simulink model "MORUS_NELINEARNI_NELINEARNI_MPC"  (R2019a)
settings: Solver=FixedStepAuto  StartTime=0.0  StopTime=sim_time  RelTol=1e-3  EnableMultiTasking=on
values from neighbouring files (symbols this model uses):
  A_dis_calc = expm(kSamplingTime*A_continous_time)    [MPC_designer_X.m]    (also in NonTilting.m; RUN_simulation.m; Simulacija_MPC_YAW_NELINEARNI.m; Simulacija_MPC_Z.m)
  B_dis_calc = integral_exp_A * B_continous_time    [MPC_designer_X.m]    (also in NonTilting.m; RUN_simulation.m; Simulacija_MPC_YAW_NELINEARNI.m; Simulacija_MPC_Z.m)
  b_f = 4.56e-4    (= 0.000456)    [LinearizacijaMatrica.m]    (also in Linearizirane_matrice.mat; MPC_designer_X.m; NonTilting.m; RUN_simulation.m)
  b_m = 0.01    [LinearizacijaMatrica.m]    (also in Linearizirane_matrice.mat; MPC_designer_X.m; NonTilting.m; RUN_simulation.m)
  BETA = 0.0    (= 0)    [LinearizacijaMatrica.m]    (also in Linearizirane_matrice.mat; MPC_designer_X.m; NonTilting.m = 0.200712863979; RUN_simulation.m)
  g = 9.80665    [LinearizacijaMatrica.m]    (also in Linearizirane_matrice.mat; MPC_designer_X.m = 9.81; NonTilting.m = 9.81; RUN_simulation.m = 9.81)
  hover = 427.6233    [MPC_designer_X.m]    (also in NonTilting.m; RUN_simulation.m; Simulacija_MPC_YAW_NELINEARNI.m; Simulacija_MPC_Z.m)
  I_b_xx = 5.5268    [MPC_designer_X.m]    (also in NonTilting.m; RUN_simulation.m; Simulacija_MPC_YAW_NELINEARNI.m; Simulacija_MPC_Z.m)
  I_b_yy = 5.5268    [MPC_designer_X.m]    (also in NonTilting.m; RUN_simulation.m; Simulacija_MPC_YAW_NELINEARNI.m; Simulacija_MPC_Z.m)
  I_b_zz = 6.8854    [MPC_designer_X.m]    (also in NonTilting.m; RUN_simulation.m; Simulacija_MPC_YAW_NELINEARNI.m; Simulacija_MPC_Z.m)
  kSamplingTime = 0.810    (= 0.81)    [MPCDesigner_YAW.m]    (also in MPC_designer_X.m = 0.1; MPC_designer_Z.m; NonTilting.m = 0.015; RUN_simulation.m = 0.015)
  L = 0.84    [LinearizacijaMatrica.m]    (also in Linearizirane_matrice.mat; MPC_designer_X.m; NonTilting.m; RUN_simulation.m)
  m = 1.0    (= 1)    [LinearizacijaMatrica.m]    (also in Linearizirane_matrice.mat; MPC_designer_X.m; NonTilting.m; RUN_simulation.m)
  M = 34.8    [LinearizacijaMatrica.m]    (also in Linearizirane_matrice.mat; MPC_designer_X.m = 34; NonTilting.m = 34; RUN_simulation.m = 34)
  m_b = 30.8    [LinearizacijaMatrica.m]    (also in Linearizirane_matrice.mat; MPC_designer_X.m; NonTilting.m; RUN_simulation.m)
  odabir = 1    [MPC_designer_X.m]    (also in NonTilting.m; RUN_simulation.m; Simulacija_MPC_YAW_NELINEARNI.m; Simulacija_MPC_Z.m)
  polu = 1.0    (= 1)    [Simulacija_Roll.m]
  Q = inv(diag([0.5800 4*kSamplingTime 0.5800 4*kSamplingTime 300 300 0.2 (0.2/3) 100 4])) * diag([0, 0, 0, 0, 0, 0, 1e5,0, 1e7, 0]) *inv(diag([0.5800 4*kSamplingTime 0.5800 4*kSamplingTime 300 300 0.2 (0.2/3.0) 100 4]))    [NonTilting.m]    (also in RUN_simulation.m = diag([ 0.135340000000000,0.002706800000000,  0.1353400, 0.00; Simulacija_MPC_YAW_NELINEARNI.m = diag([pop(5),pop(6),pop(5),pop(6), pop(7),pop(7),pop(8),pop(; Simulacija_MPC_Z.m = diag([pop(5),pop(6),pop(5),pop(6), pop(7),pop(7),pop(8),pop(; Simulacija_Roll.m = diag([pop(5),pop(6),pop(5),pop(6), pop(7),pop(7),pop(8),pop()
  R = inv(diag([0.5800 0.5800 300 300]))*diag([0, 0, 0, 0])*inv(diag([0.5800 0.5800 300 300]))    [NonTilting.m]    (also in RUN_simulation.m = diag([0.67670, 0.67670, 0.13534000, 0.13534000]); Simulacija_MPC_YAW_NELINEARNI.m = diag([pop(1),pop(1),pop(2),pop(2)]); Simulacija_MPC_Z.m = diag([pop(1),pop(1),pop(2),pop(2)]); Simulacija_Roll.m = diag([pop(1),pop(1),pop(2),pop(2)]))
  R_delta = inv(diag([0.5800 0.5800 300 300]))* diag([0,0,0,0])*inv(diag([0.5800 0.5800 300 300]))    [NonTilting.m]    (also in RUN_simulation.m = diag([0.738879858135067, 0.738879858135067, 0.00738879858135; Simulacija_MPC_YAW_NELINEARNI.m = diag([pop(3),pop(3),pop(4),pop(4)]); Simulacija_MPC_Z.m = diag([pop(3),pop(3),pop(4),pop(4)]); Simulacija_Roll.m = diag([pop(3),pop(3),pop(4),pop(4)]))
  T_r = 0.2    [LinearizacijaMatrica.m]    (also in Linearizirane_matrice.mat; MPC_designer_X.m; NonTilting.m; RUN_simulation.m)
  w_mm = 19.7845    [LinearizacijaMatrica.m]    (also in Linearizirane_matrice.mat; MPC_designer_X.m = 17; NonTilting.m = 17; RUN_simulation.m = 17)
  z_m = 0.05    [LinearizacijaMatrica.m]    (also in Linearizirane_matrice.mat; MPC_designer_X.m; NonTilting.m; RUN_simulation.m)
  z_r = 0.2    [LinearizacijaMatrica.m]    (also in Linearizirane_matrice.mat; MPC_designer_X.m; NonTilting.m; RUN_simulation.m)
  zeta_mm = 0.6544    [LinearizacijaMatrica.m]    (also in Linearizirane_matrice.mat; MPC_designer_X.m = 0.85; NonTilting.m = 0.85; RUN_simulation.m = 0.85)
libraries: simulink x6
(part 5 of 5)

== matlab function MORUS_NELINEARNI_NELINEARNI_MPC/MPC PITCH/MATLAB Function3 ==
  settings: updateMethod=DISCRETE
  data: x0_ input; u output; x_ss_ input; u_ss_ input; kreni input; A input; B input; R input; R_delta input; Q input; samplingTime input
function u    = RMSProp(x0_, x_ss_, u_ss_, kreni, A, B, R, R_delta, Q, samplingTime)

persistent new_desire_state  pred_horizon control_horizon max_iter     ...
    scale_MV_inv   scale_OV_inv gradients gradient_past ...
    x_states deriv_wrt_u epsilon delta num_heuristic_vars ...
    u_past u_current lambdas_x lambdas_u lambdas_u_ref u_horizon ref_old t u_last_step ...
    du_max u_max  rho residuum_old 

residuum = 0;


if(isempty(new_desire_state) )
    residuum_old = 1e5;
    u_last_step = zeros(4, 1);
    du_max = zeros(4,2);
    u_max = zeros(4,2);
    
    du_max(1,1) = samplingTime * 2;
    du_max(1,2) = -samplingTime * 2;
    du_max(2,1) = samplingTime * 2;
    du_max(2,2) = -samplingTime * 2;
    du_max(3,1) = 1*(samplingTime/0.01);
    du_max(3,2) = -1*(samplingTime/0.01);
    du_max(4,1) = 1*(samplingTime/0.01);
    du_max(4,2) = -1*(samplingTime/0.01);
    rho = 0.999;
    u_max(1,1) = 0.6 / 2 - 0.01;
    u_max(1,2) = -u_max(1,1);
    u_max(2,1) = 0.6 / 2 - 0.01;
    u_max(2,2) = -u_max(1,1);
    u_max(3,1) = 50;
    u_max(3,2) = -50;
    u_max(4,1) = 50;
    u_max(4,2) = -50;
    
    ref_old  = x_ss_;
    t = 0.0;
    epsilon = 0.4;
    delta = 1e-7;
    max_iter = 15;
    control_horizon = 5;
    pred_horizon = 14;
    num_heuristic_vars = 2;
    gradients = zeros(num_heuristic_vars*control_horizon,1 );
    gradient_past = zeros(num_heuristic_vars*control_horizon,1 );
    new_desire_state = true;
    scale_OV_inv = inv(diag([0.58, 4.0, 0.58, 4.0, 800, 800, 0.5236, 0.5236]));
    
    scale_MV_inv = inv(diag([0.58, 0.58, 100, 100]));
%     
%     R =diag([0.67670, 0.67670, 0.13534000, 0.13534000]);
%     R_delta = diag([0.738879858135067, 0.738879858135067, 0.007388798581351,0.007388798581351]);
%     Q = diag([ 0.135340000000000,0.002706800000000,  0.1353400, 0.002706800, 0.002706800, 0.002706800,10.7068000, 9.676700]);
%     
%     A =[    0.4271,    0.0223,         0,         0,         0,         0,         0 ,        0;
%         -8.7243,   -0.1501,         0,         0,         0,         0,         0,         0;
%         0,         0,    0.4271,    0.0223,         0,         0,         0,         0;
%         0,         0,   -8.7243,   -0.1501,         0,         0,         0,         0;
%         0,         0,         0,         0,    0.7300,         0,         0,         0;
%         0,         0,         0,         0,         0,    0.7300,         0,         0;
%         0.0090,    0.0005,    0.0090,    0.0005,    0.0001,   -0.0001,    1.0000,    0.0787;
%         0.1699,    0.0113,    0.1699,    0.0113,    0.0028,   -0.0028,         0 ,   1.0000];
%     
%     B =[ 0.5729,         0 ,        0 ,        0;
%         8.7243,         0   ,      0 ,        0;
%         0,    0.5729  ,       0 ,        0;
%         0,    8.7243 ,        0 ,        0;
%         0,         0 ,   0.2700 ,        0;
%         0,         0 ,        0 ,   0.2700;
%         -0.0037,   -0.0037,    0.0000 ,  -0.0000;
%         -0.0347,   -0.0347,    0.0005 ,  -0.0005];
    
    
    
    x_states = zeros(size(A, 1), pred_horizon+1);
    deriv_wrt_u =  zeros(size(B,2), control_horizon);
    u_past = zeros(size(B,2), 1);
    u_current = zeros(size(B,2), 1);
    u_ss_ = zeros(size(B,2), 1);
    lambdas_x = zeros(size(A, 1), pred_horizon);
    lambdas_u = zeros(size(B,2), pred_horizon);
    u_horizon = zeros(size(B,2), pred_horizon);
    lambdas_u_ref = zeros(size(B,2), pred_horizon);
    
end

residuum_signal =0.0;
residuum_state =0.0;

u = zeros(size(B,2), 1);
if(kreni ~= 3)
    return
end
x = zeros(control_horizon *num_heuristic_vars,1);
change_x = zeros(control_horizon *num_heuristic_vars,1);

if(sum(sum(abs(x_ss_ - ref_old), 'double')) < 1e-6)
    new_desire_state = false;
    
else
    new_desire_state = true;
    ref_old = x_ss_;
end
if (new_desire_state)
        new_desire_state = false;
        gradient_past = 0*gradient_past;
        residuum_old = 1e5;
end

if(residuum_old < 1e-4)
    return;
end

for iter = 1:max_iter
    x_states(:,1) = x0_ ;
    deriv_wrt_u = 0*deriv_wrt_u;
    u_past = zeros(size(B,2), 1);% u_current*1;
    
    
    
    for i = 1:pred_horizon
        if(i <= control_horizon)
            u(1,1) = x(0*control_horizon  + i);
            u(2,1) = x(0*control_horizon  + i);
            u(3,1) = x(1*control_horizon  + i);
            u(4,1) = -x(1*control_horizon  + i);
        end
        x_states(:,i+1) = A * x_states(:,i) + B * u;
        lambdas_x(:,i) = -1*x_ss_ + x_states(:,i+1);
        lambdas_u(:,i) = u - u_past;
        lambdas_u_ref(:, i) = u - u_ss_;
        
        %derivation of u
        if(i <= control_horizon)
            deriv_wrt_u(:, i) = (2*R*u) -2*R*u_ss_  + (4*R_delta*u) -2*R_delta*u_past + deriv_wrt_u(:, i) ;
            
            if(i > 1)
                deriv_wrt_u(:, i-1) = deriv_wrt_u(:, i-1) -2*R_delta*u ;
            end
        else
            deriv_wrt_u(:, control_horizon) = deriv_wrt_u(:, control_horizon) + (2*R*u) -2*R*u_ss_  + (4*R_delta*u)+ (-2*R_delta*u_past) ;
            deriv_wrt_u(:, control_horizon) = deriv_wrt_u(:, control_horizon) -2*R_delta*u ;
        end
        
        %derivation of x
        for j = 1:i
            if(j <= control_horizon && i <= control_horizon)
                
                deriv_wrt_u(:,j) = deriv_wrt_u(:,j) + transpose(transpose( 2*Q*x_states(:,i+1) - 2*Q*x_ss_ )*(A^(i-j))*B);
            else
                if(j > control_horizon)
                    deriv_wrt_u(:,control_horizon) =deriv_wrt_u(:,control_horizon) +  transpose(transpose((2*Q*x_states(:,i+1) - 2*Q*x_ss_))*(A^(i-j))*B);
                else
                    deriv_wrt_u(:,j) =deriv_wrt_u(:,j) + transpose(transpose( 2*Q*x_states(:,i+1) - 2*Q*x_ss_ )*(A^(i-j))*B);
                end
            end
        end
        u_past = u;
    end
    
    
    lambdas_u_ref =scale_MV_inv * lambdas_u_ref;
    lambdas_u = scale_MV_inv * lambdas_u;
    lambdas_x = scale_OV_inv * lambdas_x;
    residuum_signal=sum(sum((lambdas_u_ref.*(R*lambdas_u_ref)),'double'))  + sum(sum((lambdas_u.*(R_delta*lambdas_u)),'double'));
    residuum_state=sum(sum((lambdas_x.*(Q*lambdas_x)),'double')) ;
    
    residuum =  residuum_signal +  residuum_state;
    
    
    
    for iter_der = 1:control_horizon
        gradients(iter_der, 1) = 2 * deriv_wrt_u(1, iter_der);
        gradients(iter_der + control_horizon, 1) = 2 * deriv_wrt_u(3, iter_der);
    end
    
    
    gradient_past = (rho*gradient_past + (1-rho)*gradients.*gradients);
    
    
    
    for adam_iter = 1:control_horizon *num_heuristic_vars
        change_x(adam_iter, 1) = -1 * (epsilon * gradients(adam_iter, 1)) / (sqrt(gradient_past(adam_iter, 1)) + delta);
        
    end
    
    x = (x + change_x);
end

u(1,1) = x(0*control_horizon  + 1);
u(2,1) = x(0*control_horizon  + 1);
u(3,1) = x(1*control_horizon  + 1);
u(4,1) = -x(1*control_horizon  + 1);

for iter_m = 1:4
    if(u(iter_m,1) > ( u_last_step(iter_m,1)+du_max(iter_m,1) ))
        u(iter_m,1) =  u_last_step(iter_m,1)+du_max(iter_m,1);
        
    elseif (u(iter_m,1) < ( u_last_step(iter_m,1)+du_max(iter_m,2) ))
        u(iter_m,1) =  u_last_step(iter_m,1)+du_max(iter_m,2);
    end
    
    if(u(iter_m,1) > u_max(iter_m,1) )
        u(iter_m,1) =  u_max(iter_m,1);
    elseif (u(iter_m,1) < u_max(iter_m,2))
        u(iter_m,1) =  u_max(iter_m,2);
    end
    
    
end
if(residuum_old < residuum)
    u = 0*u;
    return;
end
u_last_step = u;
residuum_old = residuum;
end

== matlab function MORUS_NELINEARNI_NELINEARNI_MPC/MPC PITCH/MATLAB Function4 ==
  settings: updateMethod=DISCRETE
  data: x0_ input; u output; x_ss_ input; u_ss_ input; kreni input; A input; B input; R input; R_delta input; Q input; samplingTime input
function u   = RMSPropNester(x0_, x_ss_, u_ss_, kreni, A, B, R, R_delta, Q, samplingTime)

persistent new_desire_state  pred_horizon control_horizon max_iter    ...
    scale_MV_inv   scale_OV_inv gradients gradient_past ...
    x_states deriv_wrt_u epsilon delta num_heuristic_vars ...
    u_past u_current lambdas_x lambdas_u lambdas_u_ref u_horizon ref_old t u_last_step ...
    du_max u_max  rho residuum_old alpha change_x x

residuum = 0;


if(isempty(new_desire_state) )
    residuum_old = 1e25;
    u_last_step = zeros(4, 1);
    du_max = zeros(4,2);
    u_max = zeros(4,2);
    alpha = 200;
    du_max(1,1) = samplingTime * 2;
    du_max(1,2) = -samplingTime * 2;
    du_max(2,1) = samplingTime * 2;
    du_max(2,2) = -samplingTime * 2;
    du_max(3,1) = 1*(samplingTime/0.01);
    du_max(3,2) = -1*(samplingTime/0.01);
    du_max(4,1) = 1*(samplingTime/0.01);
    du_max(4,2) = -1*(samplingTime/0.01);
    rho = 0.999;
    u_max(1,1) = 0.6 / 2 - 0.01;
    u_max(1,2) = -u_max(1,1);
    u_max(2,1) = 0.6 / 2 - 0.01;
    u_max(2,2) = -u_max(1,1);
    u_max(3,1) = 50;
    u_max(3,2) = -50;
    u_max(4,1) = 50;
    u_max(4,2) = -50;
    
    ref_old  = x_ss_;
    t = 0.0;
    epsilon = 0.4;
    delta = 1e-7;
    max_iter = 15;
    control_horizon = 5;
    pred_horizon = 14;
    num_heuristic_vars = 2;
    gradients = zeros(num_heuristic_vars*control_horizon,1 );
    gradient_past = zeros(num_heuristic_vars*control_horizon,1 );
    new_desire_state = true;
    scale_OV_inv = inv(diag([0.58, 4.0, 0.58, 4.0, 800, 800, 0.5236, 0.5236]));
    
    scale_MV_inv = inv(diag([0.58, 0.58, 100, 100]));
    
%     R =diag([0.67670, 0.67670, 0.13534000, 0.13534000]);
%     R_delta = diag([0.738879858135067, 0.738879858135067, 0.007388798581351,0.007388798581351]);
%     Q = diag([ 0.135340000000000,0.002706800000000,  0.1353400, 0.002706800, 0.002706800, 0.002706800,10.7068000, 9.676700]);
%     
%     A =[    0.4271,    0.0223,         0,         0,         0,         0,         0 ,        0;
%         -8.7243,   -0.1501,         0,         0,         0,         0,         0,         0;
%         0,         0,    0.4271,    0.0223,         0,         0,         0,         0;
%         0,         0,   -8.7243,   -0.1501,         0,         0,         0,         0;
%         0,         0,         0,         0,    0.7300,         0,         0,         0;
%         0,         0,         0,         0,         0,    0.7300,         0,         0;
%         0.0090,    0.0005,    0.0090,    0.0005,    0.0001,   -0.0001,    1.0000,    0.0787;
%         0.1699,    0.0113,    0.1699,    0.0113,    0.0028,   -0.0028,         0 ,   1.0000];
%     
%     B =[ 0.5729,         0 ,        0 ,        0;
%         8.7243,         0   ,      0 ,        0;
%         0,    0.5729  ,       0 ,        0;
%         0,    8.7243 ,        0 ,        0;
%         0,         0 ,   0.2700 ,        0;
%         0,         0 ,        0 ,   0.2700;
%         -0.0037,   -0.0037,    0.0000 ,  -0.0000;
%         -0.0347,   -0.0347,    0.0005 ,  -0.0005];
    
    
    
    x_states = zeros(size(A, 1), pred_horizon+1);
    deriv_wrt_u =  zeros(size(B,2), control_horizon);
    u_past = zeros(size(B,2), 1);
    u_current = zeros(size(B,2), 1);
    u_ss_ = zeros(size(B,2), 1);
    lambdas_x = zeros(size(A, 1), pred_horizon);
    lambdas_u = zeros(size(B,2), pred_horizon);
    u_horizon = zeros(size(B,2), pred_horizon);
    lambdas_u_ref = zeros(size(B,2), pred_horizon);
    change_x = zeros(control_horizon *num_heuristic_vars,1);
    x = zeros(control_horizon *num_heuristic_vars,1);

    
end

residuum_signal =0.0;
residuum_state =0.0;

u = zeros(size(B,2), 1);
if(kreni ~= 4)
    return
end
change_x = zeros(control_horizon *num_heuristic_vars,1);

if(sum(sum(abs(x_ss_ - ref_old), 'double')) < 1e-6)
    new_desire_state = false;
    
else
    new_desire_state = true;
    ref_old = x_ss_;
end
if (new_desire_state)
        new_desire_state = false;
        gradient_past = 0*gradient_past;
        residuum_old = 1e25;
        alpha = 200;
        x = zeros(control_horizon *num_heuristic_vars,1);

end

if(residuum_old < 1e-4)
    return;
end

for iter = 1:max_iter
    x_states(:,1) = x0_ ;
    deriv_wrt_u = 0*deriv_wrt_u;
    u_past = zeros(size(B,2), 1);% u_current*1;
    
    
    x_tilda = x + alpha * change_x;
    for i = 1:pred_horizon
        if(i <= control_horizon)
            u(1,1) = x_tilda(0*control_horizon  + i);
            u(2,1) = x_tilda(0*control_horizon  + i);
            u(3,1) = x_tilda(1*control_horizon  + i);
            u(4,1) = -x_tilda(1*control_horizon  + i);
        end
        x_states(:,i+1) = A * x_states(:,i) + B * u;
        lambdas_x(:,i) = -1*x_ss_ + x_states(:,i+1);
        lambdas_u(:,i) = u - u_past;
        lambdas_u_ref(:, i) = u - u_ss_;
        
        %derivation of u
        if(i <= control_horizon)
            deriv_wrt_u(:, i) = (2*R*u) -2*R*u_ss_  + (4*R_delta*u) -2*R_delta*u_past + deriv_wrt_u(:, i) ;
            
            if(i > 1)
                deriv_wrt_u(:, i-1) = deriv_wrt_u(:, i-1) -2*R_delta*u ;
            end
        else
            deriv_wrt_u(:, control_horizon) = deriv_wrt_u(:, control_horizon) + (2*R*u) -2*R*u_ss_  + (4*R_delta*u)+ (-2*R_delta*u_past) ;
            deriv_wrt_u(:, control_horizon) = deriv_wrt_u(:, control_horizon) -2*R_delta*u ;
        end
        
        %derivation of x
        for j = 1:i
            if(j <= control_horizon && i <= control_horizon)
                
                deriv_wrt_u(:,j) = deriv_wrt_u(:,j) + transpose(transpose( 2*Q*x_states(:,i+1) - 2*Q*x_ss_ )*(A^(i-j))*B);
            else
                if(j > control_horizon)
                    deriv_wrt_u(:,control_horizon) =deriv_wrt_u(:,control_horizon) +  transpose(transpose((2*Q*x_states(:,i+1) - 2*Q*x_ss_))*(A^(i-j))*B);
                else
                    deriv_wrt_u(:,j) =deriv_wrt_u(:,j) + transpose(transpose( 2*Q*x_states(:,i+1) - 2*Q*x_ss_ )*(A^(i-j))*B);
                end
            end
        end
        u_past = u;
    end
    
    
    lambdas_u_ref =scale_MV_inv * lambdas_u_ref;
    lambdas_u = scale_MV_inv * lambdas_u;
    lambdas_x = scale_OV_inv * lambdas_x;
    residuum_signal=sum(sum((lambdas_u_ref.*(R*lambdas_u_ref)),'double'))  + sum(sum((lambdas_u.*(R_delta*lambdas_u)),'double'));
    residuum_state=sum(sum((lambdas_x.*(Q*lambdas_x)),'double')) ;
    
    residuum =  residuum_signal +  residuum_state;
    if(residuum < 0.1)
        alpha = 1e-5;
    end
    
    
    for iter_der = 1:control_horizon
        gradients(iter_der, 1) = 2 * deriv_wrt_u(1, iter_der);
        gradients(iter_der + control_horizon, 1) = 2 * deriv_wrt_u(3, iter_der);
    end
    
    
    gradient_past = (rho*gradient_past + (1-rho)*gradients.*gradients);
    
    
    
    for adam_iter = 1:control_horizon *num_heuristic_vars
        change_x(adam_iter, 1) =alpha * change_x(adam_iter, 1)  -1 * (epsilon * gradients(adam_iter, 1)) / (sqrt(gradient_past(adam_iter, 1)) + delta);
        
    end
    
    x = (x + change_x);
end

u(1,1) = x(0*control_horizon  + 1);
u(2,1) = x(0*control_horizon  + 1);
u(3,1) = x(1*control_horizon  + 1);
u(4,1) = -x(1*control_horizon  + 1);

for iter_m = 1:4
    if(u(iter_m,1) > ( u_last_step(iter_m,1)+du_max(iter_m,1) ))
        u(iter_m,1) =  u_last_step(iter_m,1)+du_max(iter_m,1);
        
    elseif (u(iter_m,1) < ( u_last_step(iter_m,1)+du_max(iter_m,2) ))
        u(iter_m,1) =  u_last_step(iter_m,1)+du_max(iter_m,2);
    end
    
    if(u(iter_m,1) > u_max(iter_m,1) )
        u(iter_m,1) =  u_max(iter_m,1);
    elseif (u(iter_m,1) < u_max(iter_m,2))
        u(iter_m,1) =  u_max(iter_m,2);
    end
    
    
end
if(residuum_old < residuum)
    u = 0*u;
    return;
end
u_last_step = u;
residuum_old = residuum;
end

== matlab function MORUS_NELINEARNI_NELINEARNI_MPC/MATLAB Function ==
  data: OMEGA_1 input size=1; A_dis_calc output size=8,8; OMEGA_2 input size=1; OMEGA_3 input size=1; OMEGA_4 input size=1; DOT_YAW input size=1; ROLL input size=1; PITCH input size=1; DOT_PITCH input size=1; DOT_ROLL input size=1; x_1 input size=1; x_3 input size=1; y_2 input size=1; y_4 input size=1; DOT_x_1 input size=1; DOT_x_3 input size=1; DOT_y_2 input size=1; DOT_y_4 input size=1; x_1_ref input size=1; x_3_ref input size=1; y_2_ref input size=1; y_4_ref input size=1; kSamplingTime input size=1; B_dis_calc output size=8,4
function [A_dis_calc ,B_dis_calc] = getROLLMAT(OMEGA_1, OMEGA_2, OMEGA_3, OMEGA_4, DOT_YAW , ROLL, PITCH, DOT_PITCH, DOT_ROLL,  x_1, x_3, y_2, y_4, DOT_x_1 ,DOT_x_3 ,DOT_y_2, DOT_y_4, x_1_ref, x_3_ref, y_2_ref, y_4_ref, kSamplingTime)

kGravity = 9.80665;
mass_ = 1.0;
mass_quad_ = 30.8;
M_ = mass_quad_ + 4 * mass_;
mi_ = mass_ / M_;

zm_ = 0.05;

lm_ = 0.6;
 Iq_xx = 5.5268 + 0.2;
 Iq_yy = 5.5268 + 0.2;
 Iq_zz = 6.8854 + 0.4;
Iq_ = zeros(3, 3);
Iq_(1, 1) = Iq_xx;
Iq_(2, 2) = Iq_yy;
Iq_(3, 3) = Iq_zz;
Iyy_b_ = 5.5268;
Iyy_ = Iyy_b_ + 2 * mass_ * (lm_ / 2)^ 2;

Tgm_ = 0.25;
w_gm_n_ = 7000 / 60 * 2 * pi;
F_n_ = 25 * kGravity;
b_gm_f_ = F_n_ / (w_gm_n_^ 2);

w_gm_0_ = sqrt(M_ * kGravity / 4.0 / b_gm_f_);





zeta_mm_ = 0.6544;
w_mm_ = 19.7845;
A_continous_time = zeros(8,8);
A_continous_time(1+0, 1+ 1) = 1.0;
A_continous_time(1+1, 1+ 0) = -(w_mm_^ 2);
A_continous_time(1+1, 1+ 1) = -2.0 * zeta_mm_ * w_mm_;
A_continous_time(1+2, 1+ 3) = 1.0;
A_continous_time(1+3, 1+ 2) = -(w_mm_^  2);
A_continous_time(1+3, 1+ 3) = -2.0 * zeta_mm_ * w_mm_;
A_continous_time(1+4, 1+ 4) = -1.0 / Tgm_;
A_continous_time(1+5, 1+ 5) = -1.0 / Tgm_;
A_continous_time(1+6, 1+ 7) = 1.0;
A_continous_time(1+7, 1+ 0) = 1.0 * mass_ / Iyy_ * (kGravity + ((1.0 - 4.0 * mi_) * zm_ * (w_mm_^ 2)));
A_continous_time(1+7, 1+ 1) = 2.0 * mass_ * (1.0 - 4.0 * mi_) * zm_ * zeta_mm_ * w_mm_ / Iyy_;
A_continous_time(1+7, 1+ 2) = mass_ / Iyy_ * (kGravity + ((1.0 - 4.0 * mi_) * zm_ * (w_mm_^ 2)));
A_continous_time(1+7, 1+ 3) = 2.0 * mass_ * (1.0 - 4.0 * mi_) * zm_ * zeta_mm_ * w_mm_ / Iyy_;
A_continous_time(1+7, 1+ 4) = 2 * b_gm_f_ * w_gm_0_ * lm_ / Iyy_;
A_continous_time(1+7, 1+ 5) = -2 * b_gm_f_ * w_gm_0_ * lm_ / Iyy_;

B_continous_time = zeros(8,4);
B_continous_time(1+1, 1+ 0) = (w_mm_^ 2);
B_continous_time(1+3, 1+ 1) = (w_mm_^ 2);
B_continous_time(1+4, 1+ 2) = 1.0 / Tgm_;
B_continous_time(1+5, 1+ 3) = 1.0 / Tgm_;
B_continous_time(1+7, 1+ 0) =-(16569550015242945875*cos(ROLL))/(8796093022208*(105625*x_1^2 - 6250*x_1*x_3 + 91350*x_1 + 105625*x_3^2 - 91350*x_3 + 640369));
B_continous_time(1+7, 1+ 1) =-(16569550015242945875*cos(ROLL))/(8796093022208*(105625*x_1^2 - 6250*x_1*x_3 + 91350*x_1 + 105625*x_3^2 - 91350*x_3 + 640369));


A_continous_time(8,:) = [(108750*cos(ROLL)*((3504881374004815*OMEGA_1^2)/267477789068788498432 + (3504881374004815*OMEGA_2^2)/267477789068788498432 + (3504881374004815*OMEGA_3^2)/267477789068788498432 + (3504881374004815*OMEGA_4^2)/267477789068788498432 - (14318*DOT_x_1*(DOT_PITCH*cos(ROLL) + DOT_YAW*cos(PITCH)*sin(ROLL)))/7569 + (820*DOT_x_3*(DOT_PITCH*cos(ROLL) + DOT_YAW*cos(PITCH)*sin(ROLL)))/7569 - ((5*DOT_ROLL)/174 - (5*DOT_YAW*sin(PITCH))/174)*(DOT_y_2 + DOT_y_4) - ((385*DOT_x_1)/7569 + (385*DOT_x_3)/7569)*(DOT_PITCH*cos(ROLL) + DOT_YAW*cos(PITCH)*sin(ROLL)) - (DOT_ROLL - DOT_YAW*sin(PITCH))*(DOT_PITCH*sin(ROLL) - DOT_YAW*cos(PITCH)*cos(ROLL))*((169*x_1)/87 - (5*x_3)/87 + 21/25) + 132556400121943567/7652600929320960))/(105625*x_1^2 - 6250*x_1*x_3 + 91350*x_1 + 105625*x_3^2 - 91350*x_3 + 640369) - (87000*sin(ROLL)*((5*DOT_y_2)/174 + (5*DOT_y_4)/174 + (14318*DOT_x_1*(DOT_PITCH*sin(ROLL) - DOT_YAW*cos(PITCH)*cos(ROLL)))/7569 - (820*DOT_x_3*(DOT_PITCH*sin(ROLL) - DOT_YAW*cos(PITCH)*cos(ROLL)))/7569 + ((385*DOT_x_1)/7569 + (385*DOT_x_3)/7569)*(DOT_PITCH*sin(ROLL) - DOT_YAW*cos(PITCH)*cos(ROLL)) - (DOT_ROLL - DOT_YAW*sin(PITCH))*(DOT_PITCH*cos(ROLL) + DOT_YAW*cos(PITCH)*sin(ROLL))*((169*x_1)/87 - (5*x_3)/87 + 21/25)))/(84500*x_1^2 - 5000*x_1*x_3 + 73080*x_1 + 84500*x_3^2 - 73080*x_3 + 84500*y_2^2 - 5000*y_2*y_4 + 73080*y_2 + 84500*y_4^2 - 73080*y_4 + 660417) - (7569000000*sin(ROLL)*((169*x_1)/87 - (5*x_3)/87 + 21/25)*((1345874447617849*OMEGA_2^2)/295147905179352825856 + (1345874447617849*OMEGA_4^2)/295147905179352825856 + (DOT_PITCH*sin(ROLL) - DOT_YAW*cos(PITCH)*cos(ROLL))*((820*DOT_x_1*x_3)/7569 + (820*DOT_x_3*x_1)/7569 + (820*DOT_y_2*y_4)/7569 + (820*DOT_y_4*y_2)/7569) - (DOT_PITCH*sin(ROLL) - DOT_YAW*cos(PITCH)*cos(ROLL))*((14318*DOT_x_1*x_1)/7569 + (14318*DOT_x_3*x_3)/7569 + (14318*DOT_y_2*y_2)/7569 + (14318*DOT_y_4*y_4)/7569) + (DOT_ROLL - DOT_YAW*sin(PITCH))*((77*DOT_x_1)/1740 + (77*DOT_x_3)/1740) - (DOT_PITCH*sin(ROLL) - DOT_YAW*cos(PITCH)*cos(ROLL))*((21*DOT_x_1)/25 - (21*DOT_x_3)/25 + (21*DOT_y_2)/25 - (21*DOT_y_4)/25) - (5*(x_1 + x_3)*(DOT_y_2 + DOT_y_4))/174 + (5*(y_2 + y_4)*(DOT_x_1 + DOT_x_3))/174 - (1345874447617849*OMEGA_1^2)/295147905179352825856 - (1345874447617849*OMEGA_3^2)/295147905179352825856 - ((385*(x_1 + x_3)*(DOT_x_1 + DOT_x_3))/7569 + (385*(y_2 + y_4)*(DOT_y_2 + DOT_y_4))/7569)*(DOT_PITCH*sin(ROLL) - DOT_YAW*cos(PITCH)*cos(ROLL)) + ((77*DOT_y_2)/1740 + (77*DOT_y_4)/1740)*(DOT_PITCH*cos(ROLL) + DOT_YAW*cos(PITCH)*sin(ROLL)) + (DOT_ROLL - DOT_YAW*sin(PITCH))*(DOT_PITCH*cos(ROLL) + DOT_YAW*cos(PITCH)*sin(ROLL))*((169*x_1^2)/174 - (5*x_1*x_3)/87 + (21*x_1)/25 + (169*x_3^2)/174 - (21*x_3)/25 - (169*y_2^2)/174 + (5*y_2*y_4)/87 - (21*y_2)/25 - (169*y_4^2)/174 + (21*y_4)/25)))/(84500*x_1^2 - 5000*x_1*x_3 + 73080*x_1 + 84500*x_3^2 - 73080*x_3 + 84500*y_2^2 - 5000*y_2*y_4 + 73080*y_2 + 84500*y_4^2 - 73080*y_4 + 660417)^2 - (11826562500*cos(ROLL)*((169*x_1)/87 - (5*x_3)/87 + 21/25)*((187071499653674713*DOT_x_1)/163255486492180480 + (187071499653674713*DOT_x_3)/163255486492180480 + (132556400121943567*x_1)/7652600929320960 + (132556400121943567*x_3)/7652600929320960 - (132556400121943567*x_1_ref)/7652600929320960 - (132556400121943567*x_3_ref)/7652600929320960 + (2102928824402889*OMEGA_1^2*((5*x_1)/174 + (5*x_3)/174 - 21/25))/4611686018427387904 + (2102928824402889*OMEGA_3^2*((5*x_1)/174 + (5*x_3)/174 + 21/25))/4611686018427387904 - ((5*DOT_ROLL)/174 - (5*DOT_YAW*sin(PITCH))/174)*((x_1 + x_3)*(DOT_y_2 + DOT_y_4) - (y_2 + y_4)*(DOT_x_1 + DOT_x_3)) + (3504881374004815*OMEGA_2^2*(x_1 + x_3))/267477789068788498432 + (3504881374004815*OMEGA_4^2*(x_1 + x_3))/267477789068788498432 + ((820*DOT_x_1*x_3)/7569 + (820*DOT_x_3*x_1)/7569)*(DOT_PITCH*cos(ROLL) + DOT_YAW*cos(PITCH)*sin(ROLL)) - ((14318*DOT_x_1*x_1)/7569 + (14318*DOT_x_3*x_3)/7569)*(DOT_PITCH*cos(ROLL) + DOT_YAW*cos(PITCH)*sin(ROLL)) - ((21*DOT_x_1)/25 - (21*DOT_x_3)/25)*(DOT_PITCH*cos(ROLL) + DOT_YAW*cos(PITCH)*sin(ROLL)) - ((77*DOT_y_2)/1740 + (77*DOT_y_4)/1740)*(DOT_PITCH*sin(ROLL) - DOT_YAW*cos(PITCH)*cos(ROLL)) - (DOT_ROLL - DOT_YAW*sin(PITCH))*(DOT_PITCH*sin(ROLL) - DOT_YAW*cos(PITCH)*cos(ROLL))*((169*x_1^2)/174 - (5*x_1*x_3)/87 + (21*x_1)/25 + (169*x_3^2)/174 - (21*x_3)/25 + 740609/435000) - ((385*x_1)/7569 + (385*x_3)/7569)*(DOT_PITCH*cos(ROLL) + DOT_YAW*cos(PITCH)*sin(ROLL))*(DOT_x_1 + DOT_x_3)))/(105625*x_1^2 - 6250*x_1*x_3 + 91350*x_1 + 105625*x_3^2 - 91350*x_3 + 640369)^2,
(10*sin(ROLL)*(385*DOT_ROLL + 250*y_2 + 250*y_4 - 385*DOT_YAW*sin(PITCH) - 7308*DOT_PITCH*sin(ROLL) + 7308*DOT_YAW*cos(PITCH)*cos(ROLL) - 16900*DOT_PITCH*x_1*sin(ROLL) + 500*DOT_PITCH*x_3*sin(ROLL) + 16900*DOT_YAW*x_1*cos(PITCH)*cos(ROLL) - 500*DOT_YAW*x_3*cos(PITCH)*cos(ROLL)))/(84500*x_1^2 - 5000*x_1*x_3 + 73080*x_1 + 84500*x_3^2 - 73080*x_3 + 84500*y_2^2 - 5000*y_2*y_4 + 73080*y_2 + 84500*y_4^2 - 73080*y_4 + 660417) - (108750*cos(ROLL)*((21*DOT_PITCH*cos(ROLL))/25 - (5*DOT_ROLL*y_4)/174 - (5*DOT_ROLL*y_2)/174 + (21*DOT_YAW*cos(PITCH)*sin(ROLL))/25 + (169*DOT_PITCH*x_1*cos(ROLL))/87 - (5*DOT_PITCH*x_3*cos(ROLL))/87 + (5*DOT_YAW*y_2*sin(PITCH))/174 + (5*DOT_YAW*y_4*sin(PITCH))/174 + (169*DOT_YAW*x_1*cos(PITCH)*sin(ROLL))/87 - (5*DOT_YAW*x_3*cos(PITCH)*sin(ROLL))/87 - 187071499653674713/163255486492180480))/(105625*x_1^2 - 6250*x_1*x_3 + 91350*x_1 + 105625*x_3^2 - 91350*x_3 + 640369),
(108750*cos(ROLL)*((3504881374004815*OMEGA_1^2)/267477789068788498432 + (3504881374004815*OMEGA_2^2)/267477789068788498432 + (3504881374004815*OMEGA_3^2)/267477789068788498432 + (3504881374004815*OMEGA_4^2)/267477789068788498432 + (820*DOT_x_1*(DOT_PITCH*cos(ROLL) + DOT_YAW*cos(PITCH)*sin(ROLL)))/7569 - (14318*DOT_x_3*(DOT_PITCH*cos(ROLL) + DOT_YAW*cos(PITCH)*sin(ROLL)))/7569 - ((5*DOT_ROLL)/174 - (5*DOT_YAW*sin(PITCH))/174)*(DOT_y_2 + DOT_y_4) - ((385*DOT_x_1)/7569 + (385*DOT_x_3)/7569)*(DOT_PITCH*cos(ROLL) + DOT_YAW*cos(PITCH)*sin(ROLL)) + (DOT_ROLL - DOT_YAW*sin(PITCH))*(DOT_PITCH*sin(ROLL) - DOT_YAW*cos(PITCH)*cos(ROLL))*((5*x_1)/87 - (169*x_3)/87 + 21/25) + 132556400121943567/7652600929320960))/(105625*x_1^2 - 6250*x_1*x_3 + 91350*x_1 + 105625*x_3^2 - 91350*x_3 + 640369) - (87000*sin(ROLL)*((5*DOT_y_2)/174 + (5*DOT_y_4)/174 - (820*DOT_x_1*(DOT_PITCH*sin(ROLL) - DOT_YAW*cos(PITCH)*cos(ROLL)))/7569 + (14318*DOT_x_3*(DOT_PITCH*sin(ROLL) - DOT_YAW*cos(PITCH)*cos(ROLL)))/7569 + ((385*DOT_x_1)/7569 + (385*DOT_x_3)/7569)*(DOT_PITCH*sin(ROLL) - DOT_YAW*cos(PITCH)*cos(ROLL)) + (DOT_ROLL - DOT_YAW*sin(PITCH))*(DOT_PITCH*cos(ROLL) + DOT_YAW*cos(PITCH)*sin(ROLL))*((5*x_1)/87 - (169*x_3)/87 + 21/25)))/(84500*x_1^2 - 5000*x_1*x_3 + 73080*x_1 + 84500*x_3^2 - 73080*x_3 + 84500*y_2^2 - 5000*y_2*y_4 + 73080*y_2 + 84500*y_4^2 - 73080*y_4 + 660417) + (7569000000*sin(ROLL)*((5*x_1)/87 - (169*x_3)/87 + 21/25)*((1345874447617849*OMEGA_2^2)/295147905179352825856 + (1345874447617849*OMEGA_4^2)/295147905179352825856 + (DOT_PITCH*sin(ROLL) - DOT_YAW*cos(PITCH)*cos(ROLL))*((820*DOT_x_1*x_3)/7569 + (820*DOT_x_3*x_1)/7569 + (820*DOT_y_2*y_4)/7569 + (820*DOT_y_4*y_2)/7569) - (DOT_PITCH*sin(ROLL) - DOT_YAW*cos(PITCH)*cos(ROLL))*((14318*DOT_x_1*x_1)/7569 + (14318*DOT_x_3*x_3)/7569 + (14318*DOT_y_2*y_2)/7569 + (14318*DOT_y_4*y_4)/7569) + (DOT_ROLL - DOT_YAW*sin(PITCH))*((77*DOT_x_1)/1740 + (77*DOT_x_3)/1740) - (DOT_PITCH*sin(ROLL) - DOT_YAW*cos(PITCH)*cos(ROLL))*((21*DOT_x_1)/25 - (21*DOT_x_3)/25 + (21*DOT_y_2)/25 - (21*DOT_y_4)/25) - (5*(x_1 + x_3)*(DOT_y_2 + DOT_y_4))/174 + (5*(y_2 + y_4)*(DOT_x_1 + DOT_x_3))/174 - (1345874447617849*OMEGA_1^2)/295147905179352825856 - (1345874447617849*OMEGA_3^2)/295147905179352825856 - ((385*(x_1 + x_3)*(DOT_x_1 + DOT_x_3))/7569 + (385*(y_2 + y_4)*(DOT_y_2 + DOT_y_4))/7569)*(DOT_PITCH*sin(ROLL) - DOT_YAW*cos(PITCH)*cos(ROLL)) + ((77*DOT_y_2)/1740 + (77*DOT_y_4)/1740)*(DOT_PITCH*cos(ROLL) + DOT_YAW*cos(PITCH)*sin(ROLL)) + (DOT_ROLL - DOT_YAW*sin(PITCH))*(DOT_PITCH*cos(ROLL) + DOT_YAW*cos(PITCH)*sin(ROLL))*((169*x_1^2)/174 - (5*x_1*x_3)/87 + (21*x_1)/25 + (169*x_3^2)/174 - (21*x_3)/25 - (169*y_2^2)/174 + (5*y_2*y_4)/87 - (21*y_2)/25 - (169*y_4^2)/174 + (21*y_4)/25)))/(84500*x_1^2 - 5000*x_1*x_3 + 73080*x_1 + 84500*x_3^2 - 73080*x_3 + 84500*y_2^2 - 5000*y_2*y_4 + 73080*y_2 + 84500*y_4^2 - 73080*y_4 + 660417)^2 + (11826562500*cos(ROLL)*((5*x_1)/87 - (169*x_3)/87 + 21/25)*((187071499653674713*DOT_x_1)/163255486492180480 + (187071499653674713*DOT_x_3)/163255486492180480 + (132556400121943567*x_1)/7652600929320960 + (132556400121943567*x_3)/7652600929320960 - (132556400121943567*x_1_ref)/7652600929320960 - (132556400121943567*x_3_ref)/7652600929320960 + (2102928824402889*OMEGA_1^2*((5*x_1)/174 + (5*x_3)/174 - 21/25))/4611686018427387904 + (2102928824402889*OMEGA_3^2*((5*x_1)/174 + (5*x_3)/174 + 21/25))/4611686018427387904 - ((5*DOT_ROLL)/174 - (5*DOT_YAW*sin(PITCH))/174)*((x_1 + x_3)*(DOT_y_2 + DOT_y_4) - (y_2 + y_4)*(DOT_x_1 + DOT_x_3)) + (3504881374004815*OMEGA_2^2*(x_1 + x_3))/267477789068788498432 + (3504881374004815*OMEGA_4^2*(x_1 + x_3))/267477789068788498432 + ((820*DOT_x_1*x_3)/7569 + (820*DOT_x_3*x_1)/7569)*(DOT_PITCH*cos(ROLL) + DOT_YAW*cos(PITCH)*sin(ROLL)) - ((14318*DOT_x_1*x_1)/7569 + (14318*DOT_x_3*x_3)/7569)*(DOT_PITCH*cos(ROLL) + DOT_YAW*cos(PITCH)*sin(ROLL)) - ((21*DOT_x_1)/25 - (21*DOT_x_3)/25)*(DOT_PITCH*cos(ROLL) + DOT_YAW*cos(PITCH)*sin(ROLL)) - ((77*DOT_y_2)/1740 + (77*DOT_y_4)/1740)*(DOT_PITCH*sin(ROLL) - DOT_YAW*cos(PITCH)*cos(ROLL)) - (DOT_ROLL - DOT_YAW*sin(PITCH))*(DOT_PITCH*sin(ROLL) - DOT_YAW*cos(PITCH)*cos(ROLL))*((169*x_1^2)/174 - (5*x_1*x_3)/87 + (21*x_1)/25 + (169*x_3^2)/174 - (21*x_3)/25 + 740609/435000) - ((385*x_1)/7569 + (385*x_3)/7569)*(DOT_PITCH*cos(ROLL) + DOT_YAW*cos(PITCH)*sin(ROLL))*(DOT_x_1 + DOT_x_3)))/(105625*x_1^2 - 6250*x_1*x_3 + 91350*x_1 + 105625*x_3^2 - 91350*x_3 + 640369)^2,
(10*sin(ROLL)*(385*DOT_ROLL + 250*y_2 + 250*y_4 - 385*DOT_YAW*sin(PITCH) + 7308*DOT_PITCH*sin(ROLL) - 7308*DOT_YAW*cos(PITCH)*cos(ROLL) + 500*DOT_PITCH*x_1*sin(ROLL) - 16900*DOT_PITCH*x_3*sin(ROLL) - 500*DOT_YAW*x_1*cos(PITCH)*cos(ROLL) + 16900*DOT_YAW*x_3*cos(PITCH)*cos(ROLL)))/(84500*x_1^2 - 5000*x_1*x_3 + 73080*x_1 + 84500*x_3^2 - 73080*x_3 + 84500*y_2^2 - 5000*y_2*y_4 + 73080*y_2 + 84500*y_4^2 - 73080*y_4 + 660417) + (108750*cos(ROLL)*((5*DOT_ROLL*y_2)/174 + (5*DOT_ROLL*y_4)/174 + (21*DOT_PITCH*cos(ROLL))/25 + (21*DOT_YAW*cos(PITCH)*sin(ROLL))/25 + (5*DOT_PITCH*x_1*cos(ROLL))/87 - (169*DOT_PITCH*x_3*cos(ROLL))/87 - (5*DOT_YAW*y_2*sin(PITCH))/174 - (5*DOT_YAW*y_4*sin(PITCH))/174 + (5*DOT_YAW*x_1*cos(PITCH)*sin(ROLL))/87 - (169*DOT_YAW*x_3*cos(PITCH)*sin(ROLL))/87 + 187071499653674713/163255486492180480))/(105625*x_1^2 - 6250*x_1*x_3 + 91350*x_1 + 105625*x_3^2 - 91350*x_3 + 640369),
(114346754826907089375*OMEGA_3*cos(ROLL)*((5*x_1)/174 + (5*x_3)/174 + 21/25))/(1152921504606846976*(105625*x_1^2 - 6250*x_1*x_3 + 91350*x_1 + 105625*x_3^2 - 91350*x_3 + 640369)) - (14636384617844107875*OMEGA_3*sin(ROLL))/(18446744073709551616*(84500*x_1^2 - 5000*x_1*x_3 + 73080*x_1 + 84500*x_3^2 - 73080*x_3 + 84500*y_2^2 - 5000*y_2*y_4 + 73080*y_2 + 84500*y_4^2 - 73080*y_4 + 660417)),
(114346754826907089375*OMEGA_1*cos(ROLL)*((5*x_1)/174 + (5*x_3)/174 - 21/25))/(1152921504606846976*(105625*x_1^2 - 6250*x_1*x_3 + 91350*x_1 + 105625*x_3^2 - 91350*x_3 + 640369)) - (14636384617844107875*OMEGA_1*sin(ROLL))/(18446744073709551616*(84500*x_1^2 - 5000*x_1*x_3 + 73080*x_1 + 84500*x_3^2 - 73080*x_3 + 84500*y_2^2 - 5000*y_2*y_4 + 73080*y_2 + 84500*y_4^2 - 73080*y_4 + 660417)),
(108750*cos(ROLL)*((5*DOT_YAW*cos(PITCH)*((x_1 + x_3)*(DOT_y_2 + DOT_y_4) - (y_2 + y_4)*(DOT_x_1 + DOT_x_3)))/174 - (77*DOT_YAW*cos(ROLL)*sin(PITCH)*(DOT_y_2 + DOT_y_4))/1740 - DOT_YAW*sin(PITCH)*sin(ROLL)*((820*DOT_x_1*x_3)/7569 + (820*DOT_x_3*x_1)/7569) + DOT_YAW*sin(PITCH)*sin(ROLL)*((14318*DOT_x_1*x_1)/7569 + (14318*DOT_x_3*x_3)/7569) + DOT_YAW*sin(PITCH)*sin(ROLL)*((21*DOT_x_1)/25 - (21*DOT_x_3)/25) + DOT_YAW*cos(PITCH)*(DOT_PITCH*sin(ROLL) - DOT_YAW*cos(PITCH)*cos(ROLL))*((169*x_1^2)/174 - (5*x_1*x_3)/87 + (21*x_1)/25 + (169*x_3^2)/174 - (21*x_3)/25 + 740609/435000) + DOT_YAW*sin(PITCH)*sin(ROLL)*((385*x_1)/7569 + (385*x_3)/7569)*(DOT_x_1 + DOT_x_3) - DOT_YAW*cos(ROLL)*sin(PITCH)*(DOT_ROLL - DOT_YAW*sin(PITCH))*((169*x_1^2)/174 - (5*x_1*x_3)/87 + (21*x_1)/25 + (169*x_3^2)/174 - (21*x_3)/25 + 740609/435000)))/(105625*x_1^2 - 6250*x_1*x_3 + 91350*x_1 + 105625*x_3^2 - 91350*x_3 + 640369) - (87000*sin(ROLL)*((77*DOT_YAW*cos(PITCH)*(DOT_x_1 + DOT_x_3))/1740 + DOT_YAW*cos(ROLL)*sin(PITCH)*((21*DOT_x_1)/25 - (21*DOT_x_3)/25 + (21*DOT_y_2)/25 - (21*DOT_y_4)/25) + (77*DOT_YAW*sin(PITCH)*sin(ROLL)*(DOT_y_2 + DOT_y_4))/1740 + DOT_YAW*cos(PITCH)*(DOT_PITCH*cos(ROLL) + DOT_YAW*cos(PITCH)*sin(ROLL))*((169*x_1^2)/174 - (5*x_1*x_3)/87 + (21*x_1)/25 + (169*x_3^2)/174 - (21*x_3)/25 - (21*y_2)/25 + (21*y_4)/25 + (5*y_2*y_4)/87 - (169*y_2^2)/174 - (169*y_4^2)/174) + DOT_YAW*cos(ROLL)*sin(PITCH)*((385*(x_1 + x_3)*(DOT_x_1 + DOT_x_3))/7569 + (385*(y_2 + y_4)*(DOT_y_2 + DOT_y_4))/7569) - DOT_YAW*cos(ROLL)*sin(PITCH)*((820*DOT_x_1*x_3)/7569 + (820*DOT_x_3*x_1)/7569 + (820*DOT_y_2*y_4)/7569 + (820*DOT_y_4*y_2)/7569) + DOT_YAW*cos(ROLL)*sin(PITCH)*((14318*DOT_x_1*x_1)/7569 + (14318*DOT_x_3*x_3)/7569 + (14318*DOT_y_2*y_2)/7569 + (14318*DOT_y_4*y_4)/7569) + DOT_YAW*sin(PITCH)*sin(ROLL)*(DOT_ROLL - DOT_YAW*sin(PITCH))*((169*x_1^2)/174 - (5*x_1*x_3)/87 + (21*x_1)/25 + (169*x_3^2)/174 - (21*x_3)/25 - (21*y_2)/25 + (21*y_4)/25 + (5*y_2*y_4)/87 - (169*y_2^2)/174 - (169*y_4^2)/174)))/(84500*x_1^2 - 5000*x_1*x_3 + 73080*x_1 + 84500*x_3^2 - 73080*x_3 + 84500*y_2^2 - 5000*y_2*y_4 + 73080*y_2 + 84500*y_4^2 - 73080*y_4 + 660417) + DOT_YAW*DOT_ROLL*cos(ROLL)^2*sin(PITCH) + DOT_YAW*DOT_ROLL*sin(PITCH)*sin(ROLL)^2,
- (108750*cos(ROLL)*(cos(ROLL)*((14318*DOT_x_1*x_1)/7569 + (14318*DOT_x_3*x_3)/7569) - cos(ROLL)*((820*DOT_x_1*x_3)/7569 + (820*DOT_x_3*x_1)/7569) + cos(ROLL)*((21*DOT_x_1)/25 - (21*DOT_x_3)/25) + sin(ROLL)*((77*DOT_y_2)/1740 + (77*DOT_y_4)/1740) + cos(ROLL)*((385*x_1)/7569 + (385*x_3)/7569)*(DOT_x_1 + DOT_x_3) + sin(ROLL)*(DOT_ROLL - DOT_YAW*sin(PITCH))*((169*x_1^2)/174 - (5*x_1*x_3)/87 + (21*x_1)/25 + (169*x_3^2)/174 - (21*x_3)/25 + 740609/435000)))/(105625*x_1^2 - 6250*x_1*x_3 + 91350*x_1 + 105625*x_3^2 - 91350*x_3 + 640369) - (87000*sin(ROLL)*(sin(ROLL)*((21*DOT_x_1)/25 - (21*DOT_x_3)/25 + (21*DOT_y_2)/25 - (21*DOT_y_4)/25) + sin(ROLL)*((385*(x_1 + x_3)*(DOT_x_1 + DOT_x_3))/7569 + (385*(y_2 + y_4)*(DOT_y_2 + DOT_y_4))/7569) - cos(ROLL)*((77*DOT_y_2)/1740 + (77*DOT_y_4)/1740) - sin(ROLL)*((820*DOT_x_1*x_3)/7569 + (820*DOT_x_3*x_1)/7569 + (820*DOT_y_2*y_4)/7569 + (820*DOT_y_4*y_2)/7569) + sin(ROLL)*((14318*DOT_x_1*x_1)/7569 + (14318*DOT_x_3*x_3)/7569 + (14318*DOT_y_2*y_2)/7569 + (14318*DOT_y_4*y_4)/7569) - cos(ROLL)*(DOT_ROLL - DOT_YAW*sin(PITCH))*((169*x_1^2)/174 - (5*x_1*x_3)/87 + (21*x_1)/25 + (169*x_3^2)/174 - (21*x_3)/25 - (21*y_2)/25 + (21*y_4)/25 + (5*y_2*y_4)/87 - (169*y_2^2)/174 - (169*y_4^2)/174)))/(84500*x_1^2 - 5000*x_1*x_3 + 73080*x_1 + 84500*x_3^2 - 73080*x_3 + 84500*y_2^2 - 5000*y_2*y_4 + 73080*y_2 + 84500*y_4^2 - 73080*y_4 + 660417)];




A_dis_calc = expm(kSamplingTime*A_continous_time);

count_integral_A = 10000;
integral_exp_A = 0*A_dis_calc;

%approximation of integration
for i = 1: count_integral_A
    integral_exp_A = (integral_exp_A + expm((A_continous_time * kSamplingTime * i / count_integral_A)) ...
        * kSamplingTime / count_integral_A);
end


B_dis_calc = integral_exp_A * B_continous_time;

== matlab function MORUS_NELINEARNI_NELINEARNI_MPC/DISPLAY/MATLAB Function ==
  data: v_x input; dot_p_x output; v_y input; v_z input; ROLL input; PITCH input; YAW input; dot_p_y output; dot_p_z output
function [dot_p_x,dot_p_y,dot_p_z] = fcn(v_x, v_y, v_z, ROLL, PITCH, YAW)

dot_p_x = cos(PITCH)*cos(YAW)*v_x + (sin(ROLL)*sin(PITCH)*cos(YAW) - cos(ROLL)*sin(YAW))*v_y + (cos(ROLL)*sin(PITCH)*cos(YAW) + sin(ROLL)*sin(YAW))*v_z;
dot_p_y = cos(PITCH)*sin(YAW)*v_x + (sin(ROLL)*sin(PITCH)*sin(YAW) + cos(ROLL)*cos(YAW))*v_y + (cos(ROLL)*sin(PITCH)*sin(YAW) - sin(ROLL)*cos(YAW))*v_z;
dot_p_z = -sin(PITCH)*v_x + sin(ROLL)*cos(PITCH)*v_y + cos(ROLL)*cos(PITCH)*v_z;
